simulink model "Encoder_Lab"  (R2025a)
settings: Solver=FixedStepAuto  StartTime=0.0  StopTime=inf  RelTol=1e-3  EnableMultiTasking=on
libraries: stm32g4xxblockslib x8, stm32f4xxblockslib x3
settings Model: STM32="{\"DigitalPortRead\":[{\"ID\":\"untitled:1\"},{\"ID\":\"untitled:2\"},{\"ID\":\"read_signal_ie:1\"},{\"ID\":\"read_signal_ie:2\"},{\"ID\":\"read_signal_ie:78\"}],\"EncoderBlockForG4\":[{\"ID\":\"read_signal_ie:15\"},{\"ID\":\"read_signal_ie:24\"},{\"ID\":\"read_signal_ie:29\"},{\"ID\":\"read_signal_ie:72\"},{\"ID\":\"read_signal_ie:86\"},{\"ID\":\"read_signal_ie:87\"}]}"  Creator=tawan  LastModifiedBy=tawan
settings OptimizationCC: DefaultParameterBehavior=Inlined  EnhancedBackFolding=on  PassReuseOutputArgsAs=Individual arguments  ZeroExternalMemoryAtStartup=off  ZeroInternalMemoryAtStartup=off  MaxStackSize=512  OptimizeBlockOrder=speed  DifferentSizesBufferReuse=on  OptimizationCustomize=off  EfficientTunableParamExpr=on
settings DebuggingCC: ParameterTunabilityLossMsg=error
settings HardwareCC: ProdBitPerPointer=32.0  ProdBitPerSizeT=32.0  ProdBitPerPtrDiffT=32.0  ProdLargestAtomicInteger=Long  ProdLargestAtomicFloat=Double  ProdWordSize=32.0  ProdLongLongMode=on  ProdHWDeviceType=ARM Compatible->ARM Cortex-M
settings SFSimCC: MATLABDynamicMemAlloc=off
settings RTWCC: SystemTargetFile=ert.tlc  HardwareBoard=STM32G4xx Based  TemplateMakefile=ert_default_tmf  Toolchain=GNU Tools for ARM Embedded Processors  Description=Embedded Coder
settings CodeAppCC: ForceParamTrailComments=on  IgnoreCustomStorageClasses=off  OperatorAnnotations=on  SimulinkDataObjDesc=on  SFDataObjDesc=on  InsertBlockDesc=on
settings ERTTargetCC: ExtModeTransport=3.0  ExtModeStaticAllocSize=2048.0  TargetLangStandard=C99 (ISO)  CodeReplacementLibrary=ARM Cortex-M  SupportContinuousTime=on

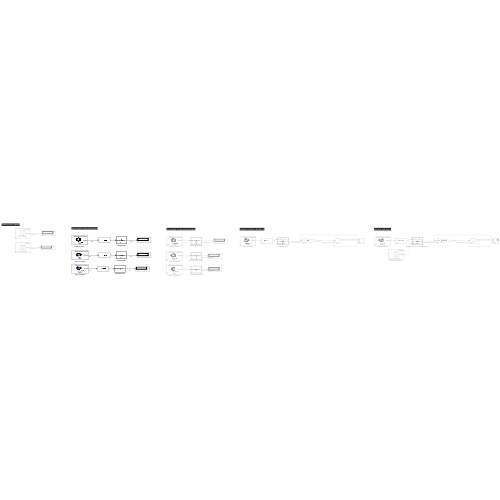
[thumbnail: Simulink's stored preview of the top-level diagram]
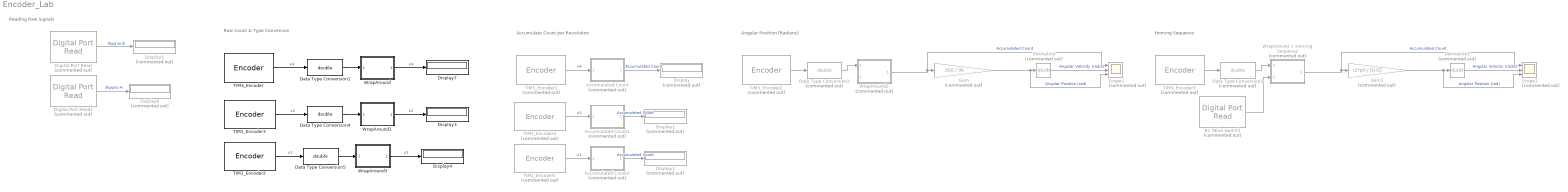
== system Encoder_Lab ==
  note: Reading Raw Signals
  note: Raw Count & Type Conversion
  note: Accumulate Count per Revolution
  note: Angular Position (Radians)
  note: Homing Sequence
  Accumulated Count : MATLAB Function  Commented=on  TreatAsAtomicUnit=on
  Accumulated Count1 : MATLAB Function  Commented=on  TreatAsAtomicUnit=on
  Accumulated Count2 : MATLAB Function  Commented=on  TreatAsAtomicUnit=on
  B1 (Blue Switch) : stm32f4xxblockslib/Digital Port Read  Commented=on  PortName=GPIOC  PinNumber=[13]  ReadOperation=on  IOAsArray=on  SampleTime=-1  EnableSimPort=off  hoistedMaskSrc=ECSoC/ECSimCodegen/Digital Port Read
  Data Type Conversion1 : DataTypeConversion  OutDataTypeStr=double  SaturateOnIntegerOverflow=off  RndMeth=Floor
  Data Type Conversion2 : DataTypeConversion  Commented=on  OutDataTypeStr=double  SaturateOnIntegerOverflow=off  RndMeth=Floor
  Data Type Conversion3 : DataTypeConversion  Commented=on  OutDataTypeStr=double  SaturateOnIntegerOverflow=off  RndMeth=Floor
  Data Type Conversion4 : DataTypeConversion  OutDataTypeStr=double  SaturateOnIntegerOverflow=off  RndMeth=Floor
  Data Type Conversion5 : DataTypeConversion  OutDataTypeStr=double  SaturateOnIntegerOverflow=off  RndMeth=Floor
  Derivative : Derivative  Commented=on
  Derivative1 : Derivative  Commented=on
  Digital Port Read : stm32f4xxblockslib/Digital Port Read  Commented=on  PortName=GPIOA  PinNumber=[6]  ReadOperation=on  IOAsArray=on  SampleTime=0.001  EnableSimPort=off  hoistedMaskSrc=ECSoC/ECSimCodegen/Digital Port Read
  Digital Port Read1 : stm32f4xxblockslib/Digital Port Read  Commented=on  PortName=GPIOA  PinNumber=[4]  ReadOperation=on  IOAsArray=on  SampleTime=0.001  EnableSimPort=off  hoistedMaskSrc=ECSoC/ECSimCodegen/Digital Port Read
  Display{,1..2,5..6} (5 alike) : Display  Commented=on
  Display3 : Display
  Display4 : Display
  Display7 : Display
  Gain : Gain  Commented=on  Gain=360 / 96  OutDataTypeStr=double
  Gain1 : Gain  Commented=on  Gain=(2*pi) / 8192  OutDataTypeStr=double
  Scope1 : Scope  Commented=on  NumInputPorts=3
  Scope2 : Scope  Commented=on  NumInputPorts=3
  TIM1_Encoder1 : stm32g4xxblockslib/Encoder  Commented=on  TimerModule=TIM4  EnableResetInput=off  OutputCountAfterFirstIndex=off  OutputValidIndex=off  OutputDirection=off  OutputStatus=off  SampleTime=-1
  TIM1_Encoder2 : stm32g4xxblockslib/Encoder  TimerModule=TIM4  EnableResetInput=off  OutputCountAfterFirstIndex=off  OutputValidIndex=off  OutputDirection=off  OutputStatus=off  SampleTime=-1
  TIM1_Encoder3 : stm32g4xxblockslib/Encoder  TimerModule=TIM1  EnableResetInput=off  OutputCountAfterFirstIndex=off  OutputValidIndex=off  OutputDirection=off  OutputStatus=off  SampleTime=-1
  TIM1_Encoder4 : stm32g4xxblockslib/Encoder  Commented=on  TimerModule=TIM1  EnableResetInput=off  OutputCountAfterFirstIndex=off  OutputValidIndex=off  OutputDirection=off  OutputStatus=off  SampleTime=-1
  TIM3_Encoder : stm32g4xxblockslib/Encoder  TimerModule=TIM3  EnableResetInput=off  OutputCountAfterFirstIndex=off  OutputValidIndex=off  OutputDirection=off  OutputStatus=off  SampleTime=-1
  TIM3_Encoder1 : stm32g4xxblockslib/Encoder  Commented=on  TimerModule=TIM3  EnableResetInput=off  OutputCountAfterFirstIndex=off  OutputValidIndex=off  OutputDirection=off  OutputStatus=off  SampleTime=-1
  TIM3_Encoder2 : stm32g4xxblockslib/Encoder  Commented=on  TimerModule=TIM3  EnableResetInput=off  OutputCountAfterFirstIndex=off  OutputValidIndex=off  OutputDirection=off  OutputStatus=off  SampleTime=-1
  TIM3_Encoder3 : stm32g4xxblockslib/Encoder  Commented=on  TimerModule=TIM3  EnableResetInput=off  OutputCountAfterFirstIndex=off  OutputValidIndex=off  OutputDirection=off  OutputStatus=off  SampleTime=-1
  WrapAround : MATLAB Function  TreatAsAtomicUnit=on
  WrapAround + Homing Sequence : MATLAB Function  Commented=on  TreatAsAtomicUnit=on
  WrapAround1 : MATLAB Function  TreatAsAtomicUnit=on
  WrapAround2 : MATLAB Function  Commented=on  TreatAsAtomicUnit=on
  WrapAround3 : MATLAB Function  TreatAsAtomicUnit=on
  wires:
  Digital Port Read/1 -> Display5/1  "สัญญาณ B"
  Digital Port Read1/1 -> Display6/1  "สัญญาณ A"
  TIM3_Encoder/1 -> Data Type Conversion1/1  "x4"
  Data Type Conversion1/1 -> WrapAround/1(current_count)
  Accumulated Count/1(accumulated_count) -> Display/1  "Accumulated Count"
  TIM3_Encoder1/1 -> Accumulated Count/1(current_count)  "x4"
  TIM3_Encoder2/1 -> Data Type Conversion2/1
  Data Type Conversion2/1 -> WrapAround2/1(current_count)
  Gain/1 -> Scope1/3, Derivative/1  "Angular Position (rad)"
  WrapAround2/1(accumulated_count) -> Scope1/1, Gain/1  "Accumulated Count"
  Derivative/1 -> Scope1/2  "Angular Velocity (rad/s)"
  WrapAround/1(accumulated_count) -> Display7/1  "x4"
  Derivative1/1 -> Scope2/2  "Angular Velocity (rad/s)"
  Data Type Conversion3/1 -> WrapAround + Homing Sequence/1(current_count)
  Gain1/1 -> Scope2/3, Derivative1/1  "Angular Position (rad)"
  WrapAround + Homing Sequence/1(accumulated_count) -> Scope2/1, Gain1/1  "Accumulated Count"
  TIM3_Encoder3/1 -> Data Type Conversion3/1
  B1 (Blue Switch)/1 -> WrapAround + Homing Sequence/2(reset_signal)
  TIM1_Encoder4/1 -> Accumulated Count1/1(current_count)  "x2"
  TIM1_Encoder1/1 -> Accumulated Count2/1(current_count)  "x1"
  Accumulated Count1/1(accumulated_count) -> Display1/1  "Accumulated Count"
  Accumulated Count2/1(accumulated_count) -> Display2/1  "Accumulated Count"
  Data Type Conversion4/1 -> WrapAround1/1(current_count)
  WrapAround1/1(accumulated_count) -> Display3/1  "x2"
  Data Type Conversion5/1 -> WrapAround3/1(current_count)
  WrapAround3/1(accumulated_count) -> Display4/1  "x1"
  TIM1_Encoder3/1 -> Data Type Conversion4/1  "x2"
  TIM1_Encoder2/1 -> Data Type Conversion5/1  "x1"

== matlab function Encoder_Lab/WrapAround ==
  data: current_count input; accumulated_count output
function accumulated_count = fcn(current_count)
%#codegen
% -------------------------------------------------------------------------
% ฟังก์ชัน Wrap-around สำหรับ Incremental Encoder
% -------------------------------------------------------------------------
% ฟังก์ชันนี้ทำหน้าที่แปลงค่า Raw Count ที่มีการวนลูป (เช่น 0-65535)
% ให้กลายเป็นค่าตำแหน่งสะสมที่เพิ่มขึ้นหรือลดลงได้อย่างต่อเนื่อง
% โดยการตรวจจับและแก้ไขปัญหา Overflow และ Underflow
%
% Input:
%   current_count: ค่า Raw Count ที่อ่านได้จาก Encoder ณ step ปัจจุบัน
%
% Output:
%   accumulated_count: ค่าตำแหน่งสะสมที่ถูกแก้ไขแล้ว
% -------------------------------------------------------------------------
% ส่วนที่ 1: การประกาศตัวแปรแบบ Persistent
% -------------------------------------------------------------------------
% 'persistent' คือคำสั่งที่ทำให้ตัวแปร "จำค่าล่าสุด" ของตัวเองไว้ได้
% แม้ว่าฟังก์ชันจะทำงานจบไปแล้วก็ตาม (เหมือน Global variable แต่ใช้ได้แค่ในฟังก์ชันนี้)
persistent last_count;      % ใช้เก็บค่า Count ของ step ที่แล้ว
persistent total_count;     % ใช้เก็บค่าตำแหน่งสะสมทั้งหมด
% -------------------------------------------------------------------------
% ส่วนที่ 2: การกำหนดค่าเริ่มต้น (Initialization)
% -------------------------------------------------------------------------
% ส่วนนี้จะทำงานแค่ "ครั้งแรกสุด" ที่ฟังก์ชันถูกเรียกใช้เท่านั้น
% เพื่อตั้งค่าเริ่มต้นให้กับตัวแปร persistent
if isempty(last_count)
last_count = current_count;  % ให้ค่าล่าสุดเริ่มต้นเท่ากับค่าปัจจุบัน
total_count = current_count; % ให้ค่าสะสมเริ่มต้นเท่ากับค่าปัจจุบัน
end
% -------------------------------------------------------------------------
% ส่วนที่ 3: ค่าคงที่ที่สำคัญ
% -------------------------------------------------------------------------
% ค่าสูงสุดของตัวนับ (Counter) ควรตั้งให้ตรงกับค่า ARR ใน STM32CubeMX
% สำหรับ Timer แบบ 16-bit ค่าสูงสุดคือ 2^16 - 1 = 65535
COUNTER_MAX = 65535;
% คำนวณค่าครึ่งหนึ่งของค่าสูงสุด เพื่อใช้เป็นเกณฑ์ในการตัดสินใจ
HALF_MAX = floor(COUNTER_MAX / 2);
% -------------------------------------------------------------------------
% ส่วนที่ 4: Logic การคำนวณและแก้ไข Overflow/Underflow
% -------------------------------------------------------------------------
% คำนวณหา "ความเปลี่ยนแปลง" จาก step ที่แล้ว
% แปลงเป็น double เพื่อให้แน่ใจว่าการลบเลขได้ผลลัพธ์ที่ถูกต้อง
delta = double(current_count) - double(last_count);
% ตรวจสอบการกระโดดของค่าที่ผิดปกติ
if delta < -HALF_MAX
% กรณี Overflow: เช่น หมุนจาก 65535 ไป 0
% ค่า delta จะกลายเป็น 0 - 65535 = -65535 ซึ่งน้อยกว่า -HALF_MAX
% เราต้องแก้ไขให้ delta กลายเป็น +1
% โดยการบวกกลับด้วยขนาดของ Counter ทั้งหมด
delta = delta + (COUNTER_MAX + 1);
elseif delta > HALF_MAX
% กรณี Underflow: เช่น หมุนจาก 0 ไป 65535
% ค่า delta จะกลายเป็น 65535 - 0 = 65535 ซึ่งมากกว่า +HALF_MAX
% เราต้องแก้ไขให้ delta กลายเป็น -1
% โดยการลบออกด้วยขนาดของ Counter ทั้งหมด
delta = delta - (COUNTER_MAX + 1);
end
% -------------------------------------------------------------------------
% ส่วนที่ 5: การอัปเดตค่าและส่งผลลัพธ์
% -------------------------------------------------------------------------
% นำค่า delta ที่ถูกต้อง มาบวกเพิ่มเข้าไปในค่าสะสมเดิม
total_count = total_count + delta;
% อัปเดตค่า 'last_count' ให้เป็นค่าปัจจุบัน เพื่อใช้ในการคำนวณรอบถัดไป
last_count = current_count;
% ส่งค่าตำแหน่งสะสมที่คำนวณได้ออกไปเป็น Output ของฟังก์ชัน
accumulated_count = total_count;
end

== matlab function Encoder_Lab/WrapAround2 ==
  data: current_count input; accumulated_count output; reset_signal input
function accumulated_count = fcn(current_count, reset_signal)
%#codegen

persistent last_count;
persistent total_count;

if isempty(last_count)
    last_count = current_count;
    total_count = current_count;
end

% --- ส่วนที่ 2.5: Logic การทำ Homing Sequence ---
if reset_signal > 0
    total_count = 0;
end

COUNTER_MAX = 65535; 
HALF_MAX = floor(COUNTER_MAX / 2);

delta = double(current_count) - double(last_count);

if delta < -HALF_MAX 
    delta = delta + (COUNTER_MAX + 1);
elseif delta > HALF_MAX
    delta = delta - (COUNTER_MAX + 1);
end

total_count = total_count + delta;
last_count = current_count;

accumulated_count = total_count;

end

== matlab function Encoder_Lab/WrapAround + Homing Sequence ==
  data: current_count input; accumulated_count output; reset_signal input
function accumulated_count = fcn(current_count, reset_signal)

persistent last_count;
persistent total_count;

if isempty(last_count)
    last_count = current_count;
    total_count = current_count;
end

% Homing Sequence
if reset_signal == 1
    total_count = 0;
end

COUNTER_MAX = 65535; 
HALF_MAX = floor(COUNTER_MAX / 2);

delta = double(current_count) - double(last_count);

if delta < -HALF_MAX 
    delta = delta + (COUNTER_MAX + 1);
elseif delta > HALF_MAX
    delta = delta - (COUNTER_MAX + 1);
end

total_count = total_count + delta;
last_count = current_count;

accumulated_count = total_count;

end

== matlab function Encoder_Lab/Accumulated Count1 ==
  data: current_count input; accumulated_count output
function accumulated_count = fcn(current_count)
%#codegen
% -------------------------------------------------------------------------
% ฟังก์ชัน Wrap-around สำหรับ Incremental Encoder
% -------------------------------------------------------------------------
% ฟังก์ชันนี้ทำหน้าที่แปลงค่า Raw Count ที่มีการวนลูป (เช่น 0-65535)
% ให้กลายเป็นค่าตำแหน่งสะสมที่เพิ่มขึ้นหรือลดลงได้อย่างต่อเนื่อง
% โดยการตรวจจับและแก้ไขปัญหา Overflow และ Underflow
%
% Input:
%   current_count: ค่า Raw Count ที่อ่านได้จาก Encoder ณ step ปัจจุบัน
%
% Output:
%   accumulated_count: ค่าตำแหน่งสะสมที่ถูกแก้ไขแล้ว
% -------------------------------------------------------------------------
% ส่วนที่ 1: การประกาศตัวแปรแบบ Persistent
% -------------------------------------------------------------------------
% 'persistent' คือคำสั่งที่ทำให้ตัวแปร "จำค่าล่าสุด" ของตัวเองไว้ได้
% แม้ว่าฟังก์ชันจะทำงานจบไปแล้วก็ตาม (เหมือน Global variable แต่ใช้ได้แค่ในฟังก์ชันนี้)
persistent last_count;      % ใช้เก็บค่า Count ของ step ที่แล้ว
persistent total_count;     % ใช้เก็บค่าตำแหน่งสะสมทั้งหมด
% -------------------------------------------------------------------------
% ส่วนที่ 2: การกำหนดค่าเริ่มต้น (Initialization)
% -------------------------------------------------------------------------
% ส่วนนี้จะทำงานแค่ "ครั้งแรกสุด" ที่ฟังก์ชันถูกเรียกใช้เท่านั้น
% เพื่อตั้งค่าเริ่มต้นให้กับตัวแปร persistent
if isempty(last_count)
last_count = current_count;  % ให้ค่าล่าสุดเริ่มต้นเท่ากับค่าปัจจุบัน
total_count = current_count; % ให้ค่าสะสมเริ่มต้นเท่ากับค่าปัจจุบัน
end
% -------------------------------------------------------------------------
% ส่วนที่ 3: ค่าคงที่ที่สำคัญ
% -------------------------------------------------------------------------
% ค่าสูงสุดของตัวนับ (Counter) ควรตั้งให้ตรงกับค่า ARR ใน STM32CubeMX
% สำหรับ Timer แบบ 16-bit ค่าสูงสุดคือ 2^16 - 1 = 65535
COUNTER_MAX = 65535;
% คำนวณค่าครึ่งหนึ่งของค่าสูงสุด เพื่อใช้เป็นเกณฑ์ในการตัดสินใจ
HALF_MAX = floor(COUNTER_MAX / 2);
% -------------------------------------------------------------------------
% ส่วนที่ 4: Logic การคำนวณและแก้ไข Overflow/Underflow
% -------------------------------------------------------------------------
% คำนวณหา "ความเปลี่ยนแปลง" จาก step ที่แล้ว
% แปลงเป็น double เพื่อให้แน่ใจว่าการลบเลขได้ผลลัพธ์ที่ถูกต้อง
delta = double(current_count) - double(last_count);
% ตรวจสอบการกระโดดของค่าที่ผิดปกติ
if delta < -HALF_MAX
% กรณี Overflow: เช่น หมุนจาก 65535 ไป 0
% ค่า delta จะกลายเป็น 0 - 65535 = -65535 ซึ่งน้อยกว่า -HALF_MAX
% เราต้องแก้ไขให้ delta กลายเป็น +1
% โดยการบวกกลับด้วยขนาดของ Counter ทั้งหมด
delta = delta + (COUNTER_MAX + 1);
elseif delta > HALF_MAX
% กรณี Underflow: เช่น หมุนจาก 0 ไป 65535
% ค่า delta จะกลายเป็น 65535 - 0 = 65535 ซึ่งมากกว่า +HALF_MAX
% เราต้องแก้ไขให้ delta กลายเป็น -1
% โดยการลบออกด้วยขนาดของ Counter ทั้งหมด
delta = delta - (COUNTER_MAX + 1);
end
% -------------------------------------------------------------------------
% ส่วนที่ 5: การอัปเดตค่าและส่งผลลัพธ์
% -------------------------------------------------------------------------
% นำค่า delta ที่ถูกต้อง มาบวกเพิ่มเข้าไปในค่าสะสมเดิม
total_count = total_count + delta;
% อัปเดตค่า 'last_count' ให้เป็นค่าปัจจุบัน เพื่อใช้ในการคำนวณรอบถัดไป
last_count = current_count;
% ส่งค่าตำแหน่งสะสมที่คำนวณได้ออกไปเป็น Output ของฟังก์ชัน
accumulated_count = total_count;
end

== matlab function Encoder_Lab/Accumulated Count2 ==
  data: current_count input; accumulated_count output
function accumulated_count = fcn(current_count)
%#codegen
% -------------------------------------------------------------------------
% ฟังก์ชัน Wrap-around สำหรับ Incremental Encoder
% -------------------------------------------------------------------------
% ฟังก์ชันนี้ทำหน้าที่แปลงค่า Raw Count ที่มีการวนลูป (เช่น 0-65535)
% ให้กลายเป็นค่าตำแหน่งสะสมที่เพิ่มขึ้นหรือลดลงได้อย่างต่อเนื่อง
% โดยการตรวจจับและแก้ไขปัญหา Overflow และ Underflow
%
% Input:
%   current_count: ค่า Raw Count ที่อ่านได้จาก Encoder ณ step ปัจจุบัน
%
% Output:
%   accumulated_count: ค่าตำแหน่งสะสมที่ถูกแก้ไขแล้ว
% -------------------------------------------------------------------------
% ส่วนที่ 1: การประกาศตัวแปรแบบ Persistent
% -------------------------------------------------------------------------
% 'persistent' คือคำสั่งที่ทำให้ตัวแปร "จำค่าล่าสุด" ของตัวเองไว้ได้
% แม้ว่าฟังก์ชันจะทำงานจบไปแล้วก็ตาม (เหมือน Global variable แต่ใช้ได้แค่ในฟังก์ชันนี้)
persistent last_count;      % ใช้เก็บค่า Count ของ step ที่แล้ว
persistent total_count;     % ใช้เก็บค่าตำแหน่งสะสมทั้งหมด
% -------------------------------------------------------------------------
% ส่วนที่ 2: การกำหนดค่าเริ่มต้น (Initialization)
% -------------------------------------------------------------------------
% ส่วนนี้จะทำงานแค่ "ครั้งแรกสุด" ที่ฟังก์ชันถูกเรียกใช้เท่านั้น
% เพื่อตั้งค่าเริ่มต้นให้กับตัวแปร persistent
if isempty(last_count)
last_count = current_count;  % ให้ค่าล่าสุดเริ่มต้นเท่ากับค่าปัจจุบัน
total_count = current_count; % ให้ค่าสะสมเริ่มต้นเท่ากับค่าปัจจุบัน
end
% -------------------------------------------------------------------------
% ส่วนที่ 3: ค่าคงที่ที่สำคัญ
% -------------------------------------------------------------------------
% ค่าสูงสุดของตัวนับ (Counter) ควรตั้งให้ตรงกับค่า ARR ใน STM32CubeMX
% สำหรับ Timer แบบ 16-bit ค่าสูงสุดคือ 2^16 - 1 = 65535
COUNTER_MAX = 65535;
% คำนวณค่าครึ่งหนึ่งของค่าสูงสุด เพื่อใช้เป็นเกณฑ์ในการตัดสินใจ
HALF_MAX = floor(COUNTER_MAX / 2);
% -------------------------------------------------------------------------
% ส่วนที่ 4: Logic การคำนวณและแก้ไข Overflow/Underflow
% -------------------------------------------------------------------------
% คำนวณหา "ความเปลี่ยนแปลง" จาก step ที่แล้ว
% แปลงเป็น double เพื่อให้แน่ใจว่าการลบเลขได้ผลลัพธ์ที่ถูกต้อง
delta = double(current_count) - double(last_count);
% ตรวจสอบการกระโดดของค่าที่ผิดปกติ
if delta < -HALF_MAX
% กรณี Overflow: เช่น หมุนจาก 65535 ไป 0
% ค่า delta จะกลายเป็น 0 - 65535 = -65535 ซึ่งน้อยกว่า -HALF_MAX
% เราต้องแก้ไขให้ delta กลายเป็น +1
% โดยการบวกกลับด้วยขนาดของ Counter ทั้งหมด
delta = delta + (COUNTER_MAX + 1);
elseif delta > HALF_MAX
% กรณี Underflow: เช่น หมุนจาก 0 ไป 65535
% ค่า delta จะกลายเป็น 65535 - 0 = 65535 ซึ่งมากกว่า +HALF_MAX
% เราต้องแก้ไขให้ delta กลายเป็น -1
% โดยการลบออกด้วยขนาดของ Counter ทั้งหมด
delta = delta - (COUNTER_MAX + 1);
end
% -------------------------------------------------------------------------
% ส่วนที่ 5: การอัปเดตค่าและส่งผลลัพธ์
% -------------------------------------------------------------------------
% นำค่า delta ที่ถูกต้อง มาบวกเพิ่มเข้าไปในค่าสะสมเดิม
total_count = total_count + delta;
% อัปเดตค่า 'last_count' ให้เป็นค่าปัจจุบัน เพื่อใช้ในการคำนวณรอบถัดไป
last_count = current_count;
% ส่งค่าตำแหน่งสะสมที่คำนวณได้ออกไปเป็น Output ของฟังก์ชัน
accumulated_count = total_count;
end

== matlab function Encoder_Lab/WrapAround1 ==
  data: current_count input; accumulated_count output
function accumulated_count = fcn(current_count)
%#codegen
% -------------------------------------------------------------------------
% ฟังก์ชัน Wrap-around สำหรับ Incremental Encoder
% -------------------------------------------------------------------------
% ฟังก์ชันนี้ทำหน้าที่แปลงค่า Raw Count ที่มีการวนลูป (เช่น 0-65535)
% ให้กลายเป็นค่าตำแหน่งสะสมที่เพิ่มขึ้นหรือลดลงได้อย่างต่อเนื่อง
% โดยการตรวจจับและแก้ไขปัญหา Overflow และ Underflow
%
% Input:
%   current_count: ค่า Raw Count ที่อ่านได้จาก Encoder ณ step ปัจจุบัน
%
% Output:
%   accumulated_count: ค่าตำแหน่งสะสมที่ถูกแก้ไขแล้ว
% -------------------------------------------------------------------------
% ส่วนที่ 1: การประกาศตัวแปรแบบ Persistent
% -------------------------------------------------------------------------
% 'persistent' คือคำสั่งที่ทำให้ตัวแปร "จำค่าล่าสุด" ของตัวเองไว้ได้
% แม้ว่าฟังก์ชันจะทำงานจบไปแล้วก็ตาม (เหมือน Global variable แต่ใช้ได้แค่ในฟังก์ชันนี้)
persistent last_count;      % ใช้เก็บค่า Count ของ step ที่แล้ว
persistent total_count;     % ใช้เก็บค่าตำแหน่งสะสมทั้งหมด
% -------------------------------------------------------------------------
% ส่วนที่ 2: การกำหนดค่าเริ่มต้น (Initialization)
% -------------------------------------------------------------------------
% ส่วนนี้จะทำงานแค่ "ครั้งแรกสุด" ที่ฟังก์ชันถูกเรียกใช้เท่านั้น
% เพื่อตั้งค่าเริ่มต้นให้กับตัวแปร persistent
if isempty(last_count)
last_count = current_count;  % ให้ค่าล่าสุดเริ่มต้นเท่ากับค่าปัจจุบัน
total_count = current_count; % ให้ค่าสะสมเริ่มต้นเท่ากับค่าปัจจุบัน
end
% -------------------------------------------------------------------------
% ส่วนที่ 3: ค่าคงที่ที่สำคัญ
% -------------------------------------------------------------------------
% ค่าสูงสุดของตัวนับ (Counter) ควรตั้งให้ตรงกับค่า ARR ใน STM32CubeMX
% สำหรับ Timer แบบ 16-bit ค่าสูงสุดคือ 2^16 - 1 = 65535
COUNTER_MAX = 65535;
% คำนวณค่าครึ่งหนึ่งของค่าสูงสุด เพื่อใช้เป็นเกณฑ์ในการตัดสินใจ
HALF_MAX = floor(COUNTER_MAX / 2);
% -------------------------------------------------------------------------
% ส่วนที่ 4: Logic การคำนวณและแก้ไข Overflow/Underflow
% -------------------------------------------------------------------------
% คำนวณหา "ความเปลี่ยนแปลง" จาก step ที่แล้ว
% แปลงเป็น double เพื่อให้แน่ใจว่าการลบเลขได้ผลลัพธ์ที่ถูกต้อง
delta = double(current_count) - double(last_count);
% ตรวจสอบการกระโดดของค่าที่ผิดปกติ
if delta < -HALF_MAX
% กรณี Overflow: เช่น หมุนจาก 65535 ไป 0
% ค่า delta จะกลายเป็น 0 - 65535 = -65535 ซึ่งน้อยกว่า -HALF_MAX
% เราต้องแก้ไขให้ delta กลายเป็น +1
% โดยการบวกกลับด้วยขนาดของ Counter ทั้งหมด
delta = delta + (COUNTER_MAX + 1);
elseif delta > HALF_MAX
% กรณี Underflow: เช่น หมุนจาก 0 ไป 65535
% ค่า delta จะกลายเป็น 65535 - 0 = 65535 ซึ่งมากกว่า +HALF_MAX
% เราต้องแก้ไขให้ delta กลายเป็น -1
% โดยการลบออกด้วยขนาดของ Counter ทั้งหมด
delta = delta - (COUNTER_MAX + 1);
end
% -------------------------------------------------------------------------
% ส่วนที่ 5: การอัปเดตค่าและส่งผลลัพธ์
% -------------------------------------------------------------------------
% นำค่า delta ที่ถูกต้อง มาบวกเพิ่มเข้าไปในค่าสะสมเดิม
total_count = total_count + delta;
% อัปเดตค่า 'last_count' ให้เป็นค่าปัจจุบัน เพื่อใช้ในการคำนวณรอบถัดไป
last_count = current_count;
% ส่งค่าตำแหน่งสะสมที่คำนวณได้ออกไปเป็น Output ของฟังก์ชัน
accumulated_count = total_count;
end

== matlab function Encoder_Lab/WrapAround3 ==
  data: current_count input; accumulated_count output
function accumulated_count = fcn(current_count)
%#codegen
% -------------------------------------------------------------------------
% ฟังก์ชัน Wrap-around สำหรับ Incremental Encoder
% -------------------------------------------------------------------------
% ฟังก์ชันนี้ทำหน้าที่แปลงค่า Raw Count ที่มีการวนลูป (เช่น 0-65535)
% ให้กลายเป็นค่าตำแหน่งสะสมที่เพิ่มขึ้นหรือลดลงได้อย่างต่อเนื่อง
% โดยการตรวจจับและแก้ไขปัญหา Overflow และ Underflow
%
% Input:
%   current_count: ค่า Raw Count ที่อ่านได้จาก Encoder ณ step ปัจจุบัน
%
% Output:
%   accumulated_count: ค่าตำแหน่งสะสมที่ถูกแก้ไขแล้ว
% -------------------------------------------------------------------------
% ส่วนที่ 1: การประกาศตัวแปรแบบ Persistent
% -------------------------------------------------------------------------
% 'persistent' คือคำสั่งที่ทำให้ตัวแปร "จำค่าล่าสุด" ของตัวเองไว้ได้
% แม้ว่าฟังก์ชันจะทำงานจบไปแล้วก็ตาม (เหมือน Global variable แต่ใช้ได้แค่ในฟังก์ชันนี้)
persistent last_count;      % ใช้เก็บค่า Count ของ step ที่แล้ว
persistent total_count;     % ใช้เก็บค่าตำแหน่งสะสมทั้งหมด
% -------------------------------------------------------------------------
% ส่วนที่ 2: การกำหนดค่าเริ่มต้น (Initialization)
% -------------------------------------------------------------------------
% ส่วนนี้จะทำงานแค่ "ครั้งแรกสุด" ที่ฟังก์ชันถูกเรียกใช้เท่านั้น
% เพื่อตั้งค่าเริ่มต้นให้กับตัวแปร persistent
if isempty(last_count)
last_count = current_count;  % ให้ค่าล่าสุดเริ่มต้นเท่ากับค่าปัจจุบัน
total_count = current_count; % ให้ค่าสะสมเริ่มต้นเท่ากับค่าปัจจุบัน
end
% -------------------------------------------------------------------------
% ส่วนที่ 3: ค่าคงที่ที่สำคัญ
% -------------------------------------------------------------------------
% ค่าสูงสุดของตัวนับ (Counter) ควรตั้งให้ตรงกับค่า ARR ใน STM32CubeMX
% สำหรับ Timer แบบ 16-bit ค่าสูงสุดคือ 2^16 - 1 = 65535
COUNTER_MAX = 65535;
% คำนวณค่าครึ่งหนึ่งของค่าสูงสุด เพื่อใช้เป็นเกณฑ์ในการตัดสินใจ
HALF_MAX = floor(COUNTER_MAX / 2);
% -------------------------------------------------------------------------
% ส่วนที่ 4: Logic การคำนวณและแก้ไข Overflow/Underflow
% -------------------------------------------------------------------------
% คำนวณหา "ความเปลี่ยนแปลง" จาก step ที่แล้ว
% แปลงเป็น double เพื่อให้แน่ใจว่าการลบเลขได้ผลลัพธ์ที่ถูกต้อง
delta = double(current_count) - double(last_count);
% ตรวจสอบการกระโดดของค่าที่ผิดปกติ
if delta < -HALF_MAX
% กรณี Overflow: เช่น หมุนจาก 65535 ไป 0
% ค่า delta จะกลายเป็น 0 - 65535 = -65535 ซึ่งน้อยกว่า -HALF_MAX
% เราต้องแก้ไขให้ delta กลายเป็น +1
% โดยการบวกกลับด้วยขนาดของ Counter ทั้งหมด
delta = delta + (COUNTER_MAX + 1);
elseif delta > HALF_MAX
% กรณี Underflow: เช่น หมุนจาก 0 ไป 65535
% ค่า delta จะกลายเป็น 65535 - 0 = 65535 ซึ่งมากกว่า +HALF_MAX
% เราต้องแก้ไขให้ delta กลายเป็น -1
% โดยการลบออกด้วยขนาดของ Counter ทั้งหมด
delta = delta - (COUNTER_MAX + 1);
end
% -------------------------------------------------------------------------
% ส่วนที่ 5: การอัปเดตค่าและส่งผลลัพธ์
% -------------------------------------------------------------------------
% นำค่า delta ที่ถูกต้อง มาบวกเพิ่มเข้าไปในค่าสะสมเดิม
total_count = total_count + delta;
% อัปเดตค่า 'last_count' ให้เป็นค่าปัจจุบัน เพื่อใช้ในการคำนวณรอบถัดไป
last_count = current_count;
% ส่งค่าตำแหน่งสะสมที่คำนวณได้ออกไปเป็น Output ของฟังก์ชัน
accumulated_count = total_count;
end

== matlab function Encoder_Lab/Accumulated Count ==
  data: current_count input; accumulated_count output
function accumulated_count = fcn(current_count)
%#codegen
% -------------------------------------------------------------------------
% ฟังก์ชัน Wrap-around สำหรับ Incremental Encoder
% -------------------------------------------------------------------------
% ฟังก์ชันนี้ทำหน้าที่แปลงค่า Raw Count ที่มีการวนลูป (เช่น 0-65535)
% ให้กลายเป็นค่าตำแหน่งสะสมที่เพิ่มขึ้นหรือลดลงได้อย่างต่อเนื่อง
% โดยการตรวจจับและแก้ไขปัญหา Overflow และ Underflow
%
% Input:
%   current_count: ค่า Raw Count ที่อ่านได้จาก Encoder ณ step ปัจจุบัน
%
% Output:
%   accumulated_count: ค่าตำแหน่งสะสมที่ถูกแก้ไขแล้ว
% -------------------------------------------------------------------------
% ส่วนที่ 1: การประกาศตัวแปรแบบ Persistent
% -------------------------------------------------------------------------
% 'persistent' คือคำสั่งที่ทำให้ตัวแปร "จำค่าล่าสุด" ของตัวเองไว้ได้
% แม้ว่าฟังก์ชันจะทำงานจบไปแล้วก็ตาม (เหมือน Global variable แต่ใช้ได้แค่ในฟังก์ชันนี้)
persistent last_count;      % ใช้เก็บค่า Count ของ step ที่แล้ว
persistent total_count;     % ใช้เก็บค่าตำแหน่งสะสมทั้งหมด
% -------------------------------------------------------------------------
% ส่วนที่ 2: การกำหนดค่าเริ่มต้น (Initialization)
% -------------------------------------------------------------------------
% ส่วนนี้จะทำงานแค่ "ครั้งแรกสุด" ที่ฟังก์ชันถูกเรียกใช้เท่านั้น
% เพื่อตั้งค่าเริ่มต้นให้กับตัวแปร persistent
if isempty(last_count)
last_count = current_count;  % ให้ค่าล่าสุดเริ่มต้นเท่ากับค่าปัจจุบัน
total_count = current_count; % ให้ค่าสะสมเริ่มต้นเท่ากับค่าปัจจุบัน
end
% -------------------------------------------------------------------------
% ส่วนที่ 3: ค่าคงที่ที่สำคัญ
% -------------------------------------------------------------------------
% ค่าสูงสุดของตัวนับ (Counter) ควรตั้งให้ตรงกับค่า ARR ใน STM32CubeMX
% สำหรับ Timer แบบ 16-bit ค่าสูงสุดคือ 2^16 - 1 = 65535
COUNTER_MAX = 65535;
% คำนวณค่าครึ่งหนึ่งของค่าสูงสุด เพื่อใช้เป็นเกณฑ์ในการตัดสินใจ
HALF_MAX = floor(COUNTER_MAX / 2);
% -------------------------------------------------------------------------
% ส่วนที่ 4: Logic การคำนวณและแก้ไข Overflow/Underflow
% -------------------------------------------------------------------------
% คำนวณหา "ความเปลี่ยนแปลง" จาก step ที่แล้ว
% แปลงเป็น double เพื่อให้แน่ใจว่าการลบเลขได้ผลลัพธ์ที่ถูกต้อง
delta = double(current_count) - double(last_count);
% ตรวจสอบการกระโดดของค่าที่ผิดปกติ
if delta < -HALF_MAX
% กรณี Overflow: เช่น หมุนจาก 65535 ไป 0
% ค่า delta จะกลายเป็น 0 - 65535 = -65535 ซึ่งน้อยกว่า -HALF_MAX
% เราต้องแก้ไขให้ delta กลายเป็น +1
% โดยการบวกกลับด้วยขนาดของ Counter ทั้งหมด
delta = delta + (COUNTER_MAX + 1);
elseif delta > HALF_MAX
% กรณี Underflow: เช่น หมุนจาก 0 ไป 65535
% ค่า delta จะกลายเป็น 65535 - 0 = 65535 ซึ่งมากกว่า +HALF_MAX
% เราต้องแก้ไขให้ delta กลายเป็น -1
% โดยการลบออกด้วยขนาดของ Counter ทั้งหมด
delta = delta - (COUNTER_MAX + 1);
end
% -------------------------------------------------------------------------
% ส่วนที่ 5: การอัปเดตค่าและส่งผลลัพธ์
% -------------------------------------------------------------------------
% นำค่า delta ที่ถูกต้อง มาบวกเพิ่มเข้าไปในค่าสะสมเดิม
total_count = total_count + delta;
% อัปเดตค่า 'last_count' ให้เป็นค่าปัจจุบัน เพื่อใช้ในการคำนวณรอบถัดไป
last_count = current_count;
% ส่งค่าตำแหน่งสะสมที่คำนวณได้ออกไปเป็น Output ของฟังก์ชัน
accumulated_count = total_count;
end
